simulink model "drone_step_response"  (R2022b)
settings: Solver=VariableStepAuto  StartTime=0.0  StopTime=20  RelTol=1e-3
settings Model: Creator=andre  LastModifiedBy=andre

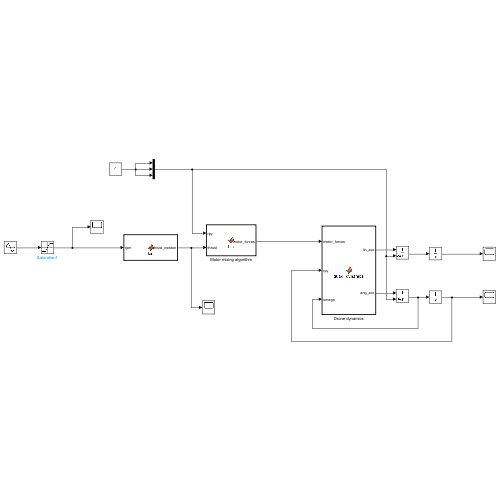
[thumbnail: Simulink's stored preview of the top-level diagram]
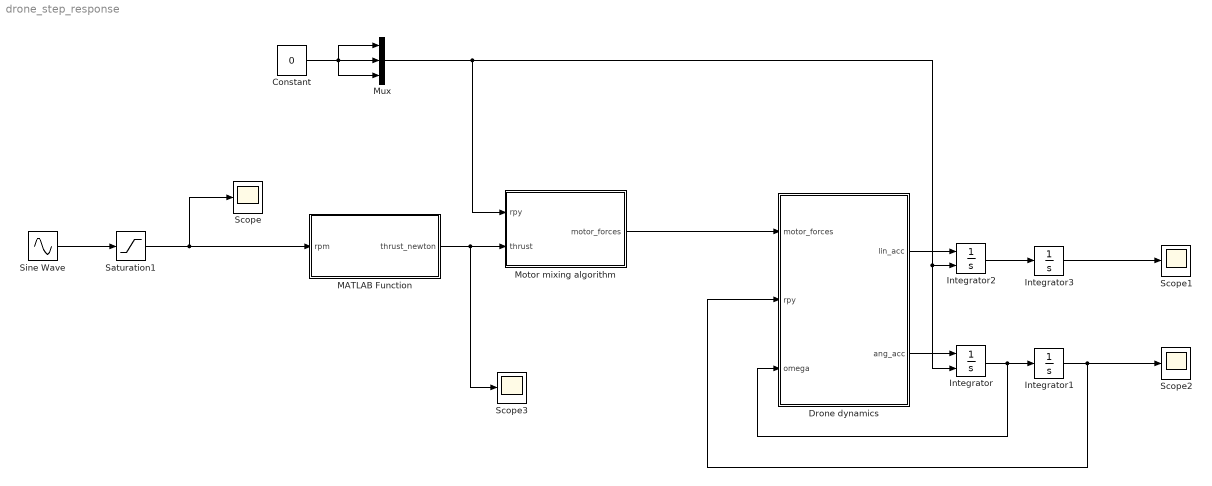
== system drone_step_response ==
  Constant : Constant  Value=0
  Drone dynamics : MATLAB Function  TreatAsAtomicUnit=on
  Integrator : Integrator  InitialConditionSource=external
  Integrator1 : Integrator
  Integrator2 : Integrator  InitialConditionSource=external
  Integrator3 : Integrator
  MATLAB Function : MATLAB Function  TreatAsAtomicUnit=on
  Motor mixing algorithm : MATLAB Function  TreatAsAtomicUnit=on
  Mux : Mux  Inputs=3
  Saturation1 : Saturate  UpperLimit=inf  LowerLimit=0
  Scope{,1..3} (4 alike) : Scope
  Sine Wave : Sin  Amplitude=17000  Frequency=0.5  SampleTime=0
  wires:
  Motor mixing algorithm/1(motor_forces) -> Drone dynamics/1(motor_forces)
  Drone dynamics/2(ang_acc) -> Integrator/1
  Integrator/1 -> Integrator1/1, Drone dynamics/3(omega)
  Integrator1/1 -> Scope2/1, Drone dynamics/2(rpy)
  Sine Wave/1 -> Saturation1/1
  MATLAB Function/1(thrust_newton) -> Scope3/1, Motor mixing algorithm/2(thrust)
  Constant/1 -> Mux/3, Mux/2, Mux/1
  Mux/1 -> Integrator2/2, Integrator/2, Motor mixing algorithm/1(rpy)
  Drone dynamics/1(lin_acc) -> Integrator2/1
  Integrator2/1 -> Integrator3/1
  Integrator3/1 -> Scope1/1
  Saturation1/1 -> MATLAB Function/1(rpm), Scope/1

== matlab function drone_step_response/Motor mixing algorithm ==
  data: motor_forces output size=[1, 4]; rpy input size=[1, 3]; thrust input
function motor_forces = fcn(rpy, thrust)

% r = rpy(1);
% p = rpy(2);
% y = rpy(3);
% 
% motor_forces = ...
% [sum([r   p   y thrust]); ...
% sum([-r   p  -y thrust]);   ...
% sum([-r  -p   y thrust]);   ...
% sum([ r  -p  -y thrust])];

m1 = thrust + rpy(1) - rpy(2) - rpy(3);
m2 = thrust - rpy(1) - rpy(2) + rpy(3);
m3 = thrust - rpy(1) + rpy(2) - rpy(3);
m4 = thrust + rpy(1) + rpy(2) + rpy(3);
motor_forces = [m1, m2, m3, m4];

== matlab function drone_step_response/Drone dynamics ==
  data: motor_forces input; lin_acc output; rpy input; ang_acc output; omega input
function [lin_acc, ang_acc] = quad_dynamics(motor_forces, rpy, omega)



%% Define constants
rotor_dist = 0.04; %m
body_mass = 0.02989; %kg
g_constant = [0;0;-9.82]; %Nm/s^2




% Vectors from CoM to motors
% We create a X-configured drone
rotor_angle = pi/4;
s1 = [cos(rotor_angle); sin(rotor_angle); 0] * rotor_dist;
s2 = [cos(rotor_angle); -sin(rotor_angle); 0] * rotor_dist;
s3 = [-cos(rotor_angle); -sin(rotor_angle); 0] * rotor_dist;
s4 = [-cos(rotor_angle); sin(rotor_angle); 0] * rotor_dist;
s_vectors = [s1 s2 s3 s4];

% Local motor force vectors
m1_vec = [0;0;motor_forces(1)];
m2_vec = [0;0;motor_forces(2)];
m3_vec = [0;0;motor_forces(3)];
m4_vec = [0;0;motor_forces(4)];
local_motor_forces = [m1_vec m2_vec m3_vec m4_vec];
    



%change the minuses if it rotates in the wrong direction, they are just
%random now
tau2m1 = [0;0;-thrust2torque(motor_forces(1))];
tau2m2 = [0;0; thrust2torque(motor_forces(2))];
tau2m3 = [0;0;-thrust2torque(motor_forces(3))];
tau2m4 = [0;0; thrust2torque(motor_forces(4))];
local_motor_torques = [tau2m1 tau2m2 tau2m3 tau2m4];

% Local inertia tensor
I_local = [1.132869584e-05 0 0; 0 1.132869584e-05 0; 0 0 2.028869584e-05];



%% Calculate drone components

% Rotation matrix
%R = rpy2r(rpy(1), rpy(2), rpy(3));
R = rotx(rpy(1)) * roty(rpy(2)) * rotz(rpy(3));

% Global inertia tensor
I_global = (R * I_local) * transpose(R);


%% Equation of motion

% Total force
total_force = R * sum(local_motor_forces,2) + (body_mass * g_constant);

% Total moment
total_moment = R * (sum(cross(s_vectors,local_motor_forces),2)+sum(local_motor_torques,2));

%% Linear and angular acceleration
a = total_force/body_mass;
lin_acc = [a(1) a(2) a(3)];

alpha = inv(I_global) * (total_moment - cross(omega,(I_global * omega)));
ang_acc = [alpha(1) alpha(2) alpha(3)];
% omega = angular velocity
% alpha = angular acceleration
end

== matlab function drone_step_response/MATLAB Function ==
  data: rpm input; thrust_newton output
function thrust_newton = fcn(rpm)

% RPM to thrust
thrust_gram = 0.109e-6*rpm^2 + -210.6e-6*rpm + 0.154;

% Gram force to Newtons
thrust_newton = thrust_gram / 101.9716212978;
